simulink model "SEIRS_meta"  (R2024a)
settings: Solver=VariableStepAuto  StartTime=0.0  StopTime=T  RelTol=1e-3
model workspace (MAT data in the model file):
  x = [0.0844291205376 0.0972801431163 0.171504041231 0.000911075297271]
values from neighbouring files (symbols this model uses):
  param_iniciales = [0.0001 0.0001 0.1 0.1 0.2 0.001]    [matlab.mat]
undefined symbols (not defined in the file or in its folder): poblacion_inicial_seirs
settings Model: Creator=carlo  LastModifiedBy=luism
settings DataIOCC: SaveOutput=off
settings RTWCC: GPUComputeCapability=3.5

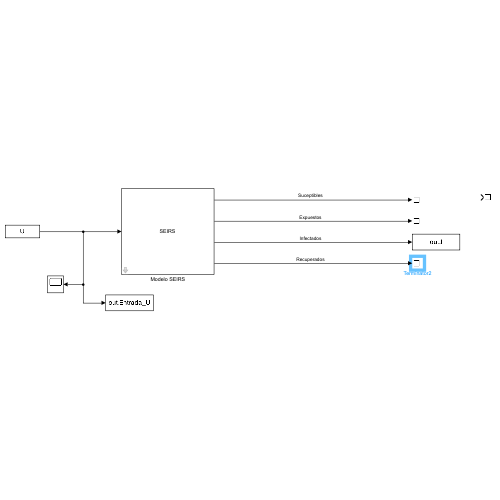
[thumbnail: Simulink's stored preview of the top-level diagram]
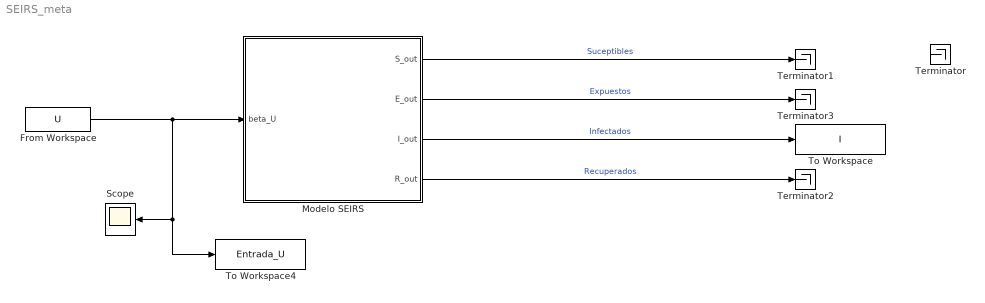
== system SEIRS_meta ==
  From Workspace : FromWorkspace  VariableName=U  SampleTime=10
  Modelo SEIRS : Subsystem  mask{B=param_iniciales(1), d=param_iniciales(2), alpha=param_iniciales(3), gamma=param_iniciales(4), beta=param_iniciales(5), nu=param_iniciales(6), ci=[poblacion_inicial_seirs(1) poblacion_inicial_seirs(2) poblacion_inicial_seirs(3) poblacion_inicial_seirs(4)], Ruido=on}
      mask prompts: ci "[S0 E0 I0 R0]"; Ruido "Incluir ruido al sistema"
      mask Display: disp('SEIRS');
  Scope : Scope
  Terminator{,1..3} (4 alike) : Terminator
  To Workspace : ToWorkspace  VariableName=I  SaveFormat=Structure With Time  SampleTime=10
  To Workspace4 : ToWorkspace  VariableName=Entrada_U  SaveFormat=Structure With Time  SampleTime=10
  wires:
  From Workspace/1 -> Scope/1, To Workspace4/1, Modelo SEIRS/1(beta_U)
  Modelo SEIRS/2(E_out) -> Terminator3/1  "Expuestos"
  Modelo SEIRS/3("I_out ") -> To Workspace/1  "Infectados"
  Modelo SEIRS/1(S_out) -> Terminator1/1  "Suceptibles"
  Modelo SEIRS/4(R_out) -> Terminator2/1  "Recuperados"

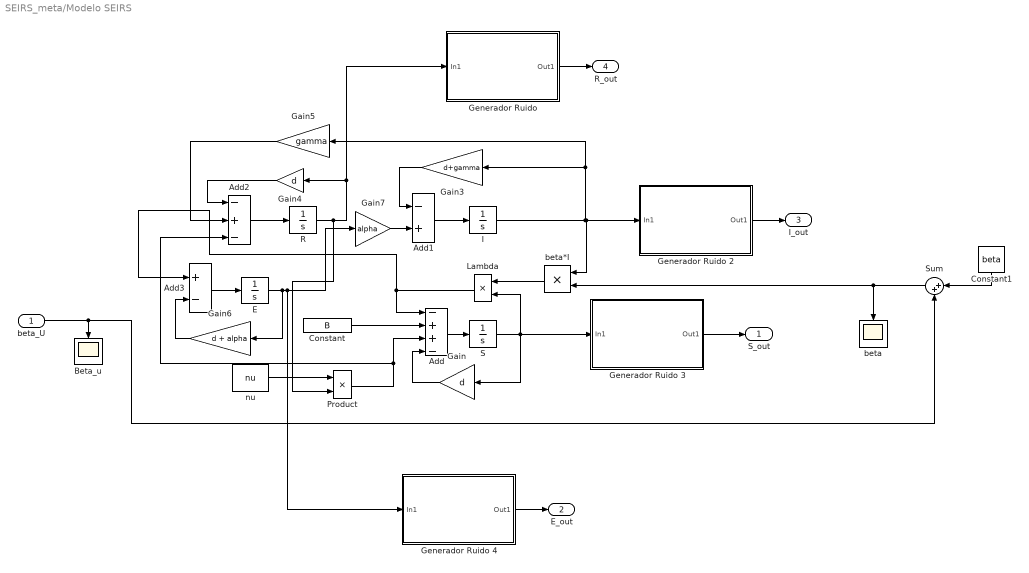
== system SEIRS_meta/Modelo SEIRS ==
  beta_U : Inport
  Add : Sum  Inputs=-++-
  Add1 : Sum  Inputs=-+
  Add2 : Sum  Inputs=-+-
  Add3 : Sum  Inputs=+-
  Beta_u : Scope
  Constant : Constant  Value=B
  Constant1 : Constant  Value=beta
  E : Integrator  InitialCondition=ci(2)  LimitOutput=on  LowerSaturationLimit=0
  Gain : Gain  Gain=d
  Gain3 : Gain  Gain=d+gamma
  Gain4 : Gain  Gain=d
  Gain5 : Gain  Gain=gamma
  Gain6 : Gain  Gain=d + alpha
  Gain7 : Gain  Gain=alpha
  "Generador Ruido " : Subsystem
      mask Display: disp('Generador Ruido');
  Generador Ruido 2 : Subsystem
      mask Display: disp('Generador Ruido');
  Generador Ruido 3 : Subsystem
      mask Display: disp('Generador Ruido');
  Generador Ruido 4 : Subsystem
      mask Display: disp('Generador Ruido');
  I : Integrator  InitialCondition=ci(3)  LimitOutput=on  LowerSaturationLimit=0
  Lambda : Product
  Product : Product
  R : Integrator  InitialCondition=ci(4)  LimitOutput=on  LowerSaturationLimit=0
  S : Integrator  InitialCondition=ci(1)  LimitOutput=on  LowerSaturationLimit=0
  Sum : Sum  Inputs=|++
  beta : Scope
  beta*I : Product
  nu : Constant  Value=nu
  S_out : Outport
  E_out : Outport  Port=2
  "I_out " : Outport  Port=3
  R_out : Outport  Port=4
  wires:
  Gain/1 -> Add/4
  Gain4/1 -> Add2/1
  Constant/1 -> Add/2
  I/1 -> Generador Ruido 2/1(In1), beta*I/1, Gain5/1, Gain3/1
  Lambda/1 -> Add3/1, Add/1
  Add/1 -> S/1
  E/1 -> Gain7/1, Generador Ruido 4/1(In1), Gain6/1
  S/1 -> Generador Ruido 3/1(In1), Lambda/2, Gain/1
  Add3/1 -> E/1
  Gain3/1 -> Add1/1
  Gain5/1 -> Add2/2
  Gain6/1 -> Add3/2
  Add1/1 -> I/1
  R/1 -> "Generador Ruido "/1(In1), Gain4/1, Product/2
  Add2/1 -> R/1
  Product/1 -> Add2/3, Add/3
  Gain7/1 -> Add1/2
  nu/1 -> Product/1
  beta*I/1 -> Lambda/1
  Sum/1 -> beta*I/2, beta/1
  Constant1/1 -> Sum/1
  beta_U/1 -> Sum/2, Beta_u/1
  Generador Ruido 2/1(Out1) -> "I_out "/1
  "Generador Ruido "/1(Out1) -> R_out/1
  Generador Ruido 3/1(Out1) -> S_out/1
  Generador Ruido 4/1(Out1) -> E_out/1

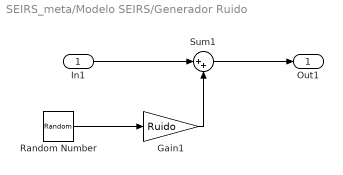
== system SEIRS_meta/Modelo SEIRS/Generador Ruido  ==
  In1 : Inport
  Gain1 : Gain  Gain=Ruido
  Random Number : RandomNumber  Variance=1e-9  Seed=117  SampleTime=0.1
  Sum1 : Sum  Inputs=|++
  Out1 : Outport
  wires:
  Random Number/1 -> Gain1/1
  Gain1/1 -> Sum1/2
  In1/1 -> Sum1/1
  Sum1/1 -> Out1/1

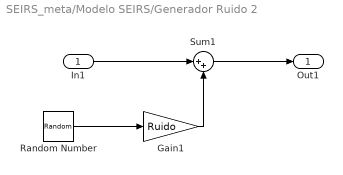
== system SEIRS_meta/Modelo SEIRS/Generador Ruido 2 ==
  In1 : Inport
  Gain1 : Gain  Gain=Ruido
  Random Number : RandomNumber  Variance=1e-7  Seed=117  SampleTime=0.1
  Sum1 : Sum  Inputs=|++
  Out1 : Outport
  wires:
  Random Number/1 -> Gain1/1
  Gain1/1 -> Sum1/2
  In1/1 -> Sum1/1
  Sum1/1 -> Out1/1

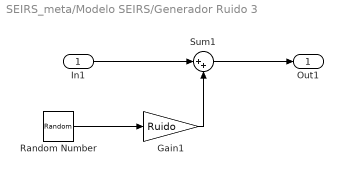
== system SEIRS_meta/Modelo SEIRS/Generador Ruido 3 ==
  In1 : Inport
  Gain1 : Gain  Gain=Ruido
  Random Number : RandomNumber  Variance=1e-9  Seed=117  SampleTime=0.1
  Sum1 : Sum  Inputs=|++
  Out1 : Outport
  wires:
  Random Number/1 -> Gain1/1
  Gain1/1 -> Sum1/2
  In1/1 -> Sum1/1
  Sum1/1 -> Out1/1

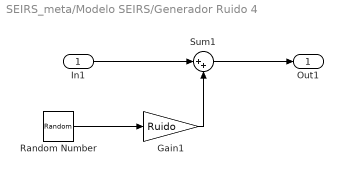
== system SEIRS_meta/Modelo SEIRS/Generador Ruido 4 ==
  In1 : Inport
  Gain1 : Gain  Gain=Ruido
  Random Number : RandomNumber  Variance=1e-9  Seed=117  SampleTime=0.1
  Sum1 : Sum  Inputs=|++
  Out1 : Outport
  wires:
  Random Number/1 -> Gain1/1
  Gain1/1 -> Sum1/2
  In1/1 -> Sum1/1
  Sum1/1 -> Out1/1
